simulink model "P2a_PI_design"  (Simulink 7.9)
settings: Solver=ode45  StartTime=0.0  StopTime=1600  RelTol=1e-3
undefined symbols (not defined in the file): beta, c1, c2
libraries: simulink x1
settings Model: Creator=matias  LastModifiedBy=matias

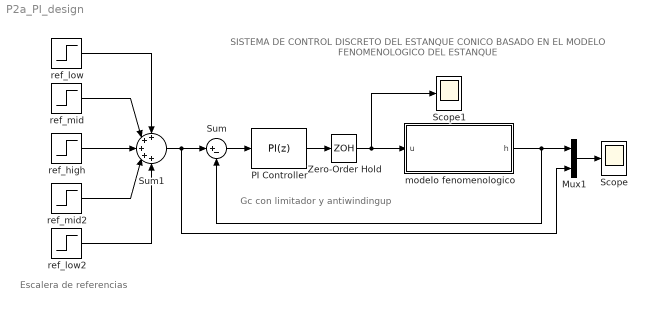
== system P2a_PI_design ==
  note: Escalera de referencias
  note: SISTEMA DE CONTROL DISCRETO DEL ESTANQUE CONICO
      | BASADO EN EL MODELO FENOMENOLOGICO DEL ESTANQUE
  note: Gc con limitador y antiwindingup
  Mux1 : Mux  Inputs=2
  PI Controller : simulink/Continuous/PID Controller  Controller=PI  TimeDomain=Discrete-time  SampleTime=1  IntegratorMethod=Forward Euler  FilterMethod=Forward Euler  Form=Parallel  P=100  I=0.05  D=0  N=100  InitialConditionSource=internal  InitialConditionForIntegrator=0  InitialConditionForFilter=0  ExternalReset=none  LimitOutput=on  UpperSaturationLimit=100  LowerSaturationLimit=0  LinearizeAsGain=off  AntiWindupMode=clamping  Kb=1  TrackingMode=off  Kt=1  PParamMin=[]  PParamMax=[]  IParamMin=[]  IParamMax=[]  DParamMin=[]  DParamMax=[]  NParamMin=[]  NParamMax=[]  KbParamMin=[]  KbParamMax=[]  KtParamMin=[]  KtParamMax=[]  POutMin=[]  POutMax=[]  IOutMin=[]  IOutMax=[]  DOutMin=[]  DOutMax=[]  NOutMin=[]  NOutMax=[]  KbOutMin=[]  KbOutMax=[]  KtOutMin=[]  KtOutMax=[]  IntegratorOutMin=[]  IntegratorOutMax=[]  FilterOutMin=[]  FilterOutMax=[]  SumOutMin=[]  SumOutMax=[]  SumI1OutMin=[]  SumI1OutMax=[]  SumI2OutMin=[]  SumI2OutMax=[]  SumI3OutMin=[]  SumI3OutMax=[]  SumDOutMin=[]  SumDOutMax=[]  SaturationOutMin=[]  SaturationOutMax=[]  IntegratorContinuousStateAttributes=''  IntegratorStateMustResolveToSignalObject=off  IntegratorRTWStateStorageClass=Auto  FilterContinuousStateAttributes=''  FilterStateMustResolveToSignalObject=off  FilterRTWStateStorageClass=Auto
  Scope : Scope
      settings: TimeRange=1600  YMin=0  YMax=60
  Scope1 : Scope
  Sum : Sum  Inputs=|+-
  Sum1 : Sum  Inputs=+++++
  Zero-Order Hold : ZeroOrderHold
  modelo fenomenologico : Subsystem  Tag=Modelo Fenomenologico
  ref_high : Step  Time=600  After=52.5-37.5  SampleTime=0
  ref_low : Step  Time=0  After=22.5  SampleTime=0
  ref_low2 : Step  Time=1200  After=22.5 - 37.5  SampleTime=0
  ref_mid : Step  Time=200  After=37.5-22.5  SampleTime=0
  ref_mid2 : Step  Time=800  After=37.5-52.5  SampleTime=0
  wires:
  Sum1/1 -> Sum/1, Mux1/2
  Sum/1 -> PI Controller/1
  modelo fenomenologico/1(h) -> Sum/2, Mux1/1
  PI Controller/1 -> Zero-Order Hold/1
  Mux1/1 -> Scope/1
  ref_high/1 -> Sum1/3
  ref_mid/1 -> Sum1/2
  ref_low/1 -> Sum1/1
  ref_mid2/1 -> Sum1/4
  ref_low2/1 -> Sum1/5
  Zero-Order Hold/1 -> modelo fenomenologico/1(u), Scope1/1

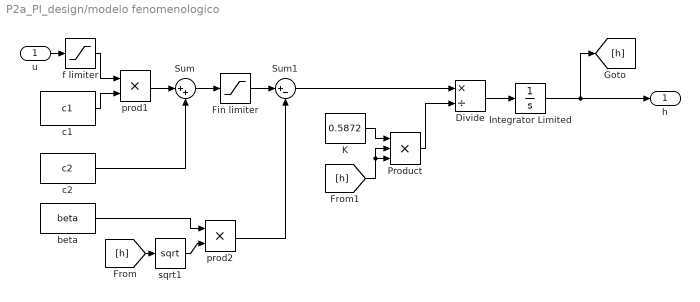
== system P2a_PI_design/modelo fenomenologico ==
  u : Inport
  Divide : Product  Inputs=*/
  Fin limiter : Saturate  UpperLimit=inf  LowerLimit=0
  Integrator Limited : Integrator  InitialCondition=0.1  LimitOutput=on  UpperSaturationLimit=80  LowerSaturationLimit=0.1
  K : Constant  Value=0.5872
  Product : Product  Inputs=3  RndMeth=Zero
  Sum : Sum  Inputs=|++
  Sum1 : Sum  Inputs=|+-
  beta : Constant  Value=beta
  c1 : Constant  Value=c1
  c2 : Constant  Value=c2
  f limiter : Saturate  UpperLimit=100  LowerLimit=0
  prod1 : Product  RndMeth=Zero
  prod2 : Product  RndMeth=Zero
  sqrt1 : Sqrt  SaturateOnIntegerOverflow=on
  h : Outport
  wires:
  f limiter/1 -> prod1/1
  c1/1 -> prod1/2
  prod1/1 -> Sum/1
  c2/1 -> Sum/2
  beta/1 -> prod2/1
  prod2/1 -> Sum1/2
  sqrt1/1 -> prod2/2
  Sum1/1 -> Divide/1
  [h] -> sqrt1/1
  Product/1 -> Divide/2
  K/1 -> Product/1
  [h] -> Product/2, Product/3
  Divide/1 -> Integrator Limited/1
  Integrator Limited/1 -> h/1, [h]
  Sum/1 -> Fin limiter/1
  Fin limiter/1 -> Sum1/1
  u/1 -> f limiter/1
